simulink model "SYS5100_Project_Simulink_Model_Group4"  (R2022a)
settings: Solver=VariableStepAuto  StartTime=0.0  StopTime=100  RelTol=1e-3
settings Model: Creator=hp  LastModifiedBy=VIKRAM
settings DebuggingCC: UnconnectedInputMsg=warning  UnconnectedOutputMsg=warning  UnconnectedLineMsg=warning
settings RTWCC: DLArmComputeVersion=19.05

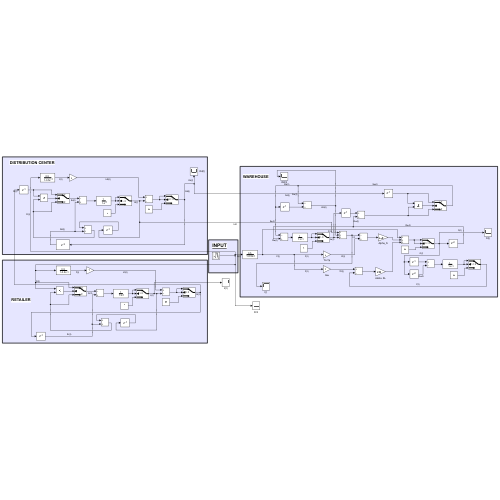
[thumbnail: Simulink's stored preview of the top-level diagram]
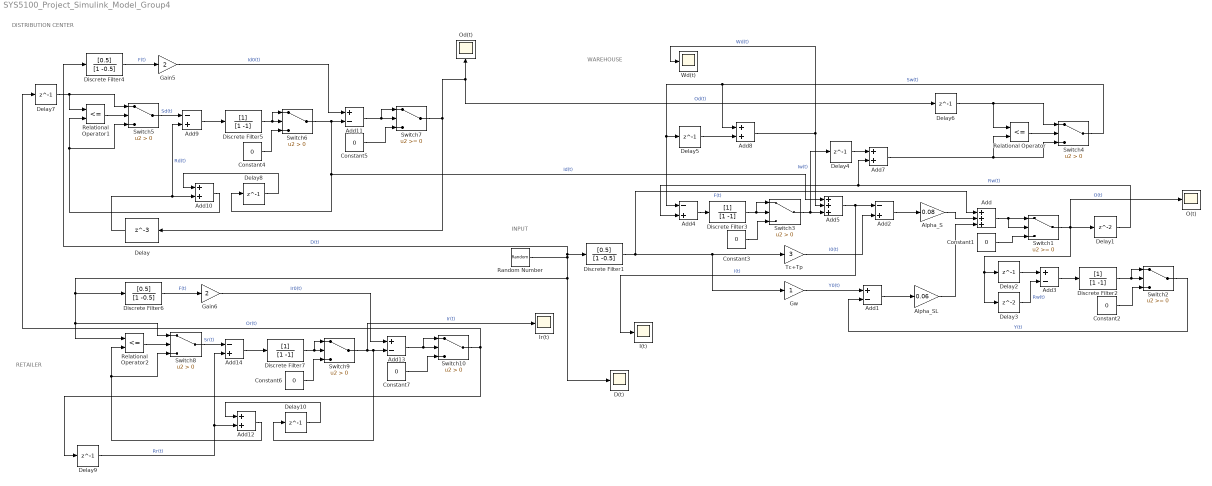
== system SYS5100_Project_Simulink_Model_Group4 ==
  note: WAREHOUSE
  note: INPUT
  note: DISTRIBUTION CENTER
  note: RETAILER
  Add : Sum  Inputs=+++
  Add{1,3,11,13} (4 alike) : Sum  Inputs=+-
  Add{7..8,10,12} (4 alike) : Sum
  Add{2,4,9,14} (4 alike) : Sum  Inputs=-+
  Add5 : Sum  Inputs=+++
  Alpha_S : Gain  Gain=0.08
  Alpha_SL : Gain  Gain=0.06
  Constant{1..7} (7 alike) : Constant  Value=0
  D(t) : Scope
  Delay : Delay  DelayLength=3  InputProcessing=Columns as channels (frame based)
  Delay1 : Delay  InitialCondition=0
  Delay{2,4..10} (8 alike) : Delay  DelayLength=1  InitialCondition=0
  Delay3 : Delay  InitialCondition=0
  Discrete Filter1 : DiscreteFilter  Numerator=[0.5]  Denominator=[1 -0.5]
  Discrete Filter{2..3,5,7} (4 alike) : DiscreteFilter  Denominator=[1 -1]
  Discrete Filter4 : DiscreteFilter  Numerator=[0.5]  Denominator=[1 -0.5]
  Discrete Filter6 : DiscreteFilter  Numerator=[0.5]  Denominator=[1 -0.5]
  Gain5 : Gain  Gain=2
  Gain6 : Gain  Gain=2
  Gw : Gain
  I(t) : Scope
  Ir(t) : Scope
  O(t) : Scope
  Od(t) : Scope
  Random Number : RandomNumber  Mean=500  Variance=100  SampleTime=1
  Relational Operator : RelationalOperator  Operator=<=  OutDataTypeStr=boolean  RndMeth=Simplest  InputSameDT=off
  Relational Operator1 : RelationalOperator  Operator=<=  OutDataTypeStr=boolean  RndMeth=Simplest  InputSameDT=off
  Relational Operator2 : RelationalOperator  Operator=<=  OutDataTypeStr=boolean  RndMeth=Simplest  InputSameDT=off
  Switch1 : Switch  SaturateOnIntegerOverflow=off  InputSameDT=off
  Switch{3..6,8..10} (7 alike) : Switch  Criteria=u2 > Threshold  SaturateOnIntegerOverflow=off  InputSameDT=off
  Switch2 : Switch  SaturateOnIntegerOverflow=off  InputSameDT=off
  Switch7 : Switch  SaturateOnIntegerOverflow=off  InputSameDT=off
  Tc+Tp : Gain  Gain=3
  Wd(t) : Scope
  wires:
  Discrete Filter1/1 -> Add/1, Gw/1, Tc+Tp/1  "F(t)"
  Gw/1 -> Add1/1  "Y0(t)"
  Tc+Tp/1 -> Add2/2  "I0(t)"
  Add2/1 -> Alpha_S/1
  Add1/1 -> Alpha_SL/1
  Alpha_S/1 -> Add/2
  Alpha_SL/1 -> Add/3
  Add/1 -> Switch1/2, Switch1/1
  Constant1/1 -> Switch1/3
  Switch1/1 -> O(t)/1, Delay3/1, Delay2/1, Delay1/1  "O(t)"
  Delay2/1 -> Add3/1
  Delay3/1 -> Add3/2  "Rw(t)"
  Add3/1 -> Discrete Filter2/1
  Discrete Filter2/1 -> Switch2/1, Switch2/2
  Constant2/1 -> Switch2/3
  Switch2/1 -> Add1/2  "Y(t)"
  Constant3/1 -> Switch3/3
  Discrete Filter3/1 -> Switch3/1, Switch3/2
  Add4/1 -> Discrete Filter3/1
  Switch3/1 -> Add5/3, Delay4/1  "Iw(t)"
  Delay1/1 -> Add7/2, Add4/2  "Rw(t)"
  Add5/1 -> I(t)/1, Add2/1  "I(t)"
  Delay4/1 -> Add7/1
  Delay5/1 -> Add8/2
  Relational Operator/1 -> Switch4/2
  Delay6/1 -> Switch4/1, Relational Operator/1
  Random Number/1 -> D(t)/1, Relational Operator2/1, Switch8/1, Discrete Filter6/1, Discrete Filter1/1, Discrete Filter4/1  "D(t)"
  Add8/1 -> Wd(t)/1, Add5/2  "Wd(t)"
  Add7/1 -> Relational Operator/2, Switch4/3
  Switch4/1 -> Add8/1, Add4/1, Delay5/1  "Sw(t)"
  Switch6/1 -> Add5/1, Delay8/1, Add11/2  "Id(t)"
  Discrete Filter4/1 -> Gain5/1  "F(t)"
  Relational Operator1/1 -> Switch5/2
  Delay7/1 -> Relational Operator1/1, Switch5/1
  Switch5/1 -> Add9/1  "Sd(t)"
  Add9/1 -> Discrete Filter5/1
  Discrete Filter5/1 -> Switch6/1, Switch6/2
  Constant4/1 -> Switch6/3
  Delay8/1 -> Add10/1
  Gain5/1 -> Add11/1  "Id0(t)"
  Delay/1 -> Add9/2, Add10/2  "Rd(t)"
  Add10/1 -> Switch5/3, Relational Operator1/2
  Add11/1 -> Switch7/1, Switch7/2
  Switch7/1 -> Delay/1, Od(t)/1, Delay6/1  "Od(t)"
  Constant5/1 -> Switch7/3
  Relational Operator2/1 -> Switch8/2
  Delay9/1 -> Add14/2, Add12/2  "Rr(t)"
  Constant7/1 -> Switch10/3
  Constant6/1 -> Switch9/3
  Switch9/1 -> Ir(t)/1, Delay10/1, Add13/2  "Ir(t)"
  Add13/1 -> Switch10/1, Switch10/2
  Gain6/1 -> Add13/1  "Ir0(t)"
  Discrete Filter7/1 -> Switch9/1, Switch9/2
  Discrete Filter6/1 -> Gain6/1  "F(t)"
  Add14/1 -> Discrete Filter7/1
  Add12/1 -> Switch8/3, Relational Operator2/2
  Delay10/1 -> Add12/1
  Switch8/1 -> Add14/1  "Sr(t)"
  Switch10/1 -> Delay9/1, Delay7/1  "Or(t)"
